simulink model "ABS_Simulink_Model"  (R2023b)
settings: Solver=VariableStepAuto  StartTime=0.0  StopTime=20  RelTol=1e-3
undefined symbols (not defined in the file): A, B, Brake_factor, C, Ch, D, g, I, mv, Rh, Rw, v0
libraries: slpidlib x1
settings Model: Creator=C837312043  LastModifiedBy=C837312043

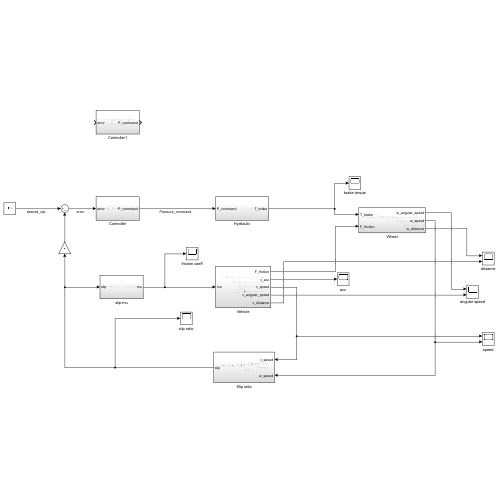
[thumbnail: Simulink's stored preview of the top-level diagram]
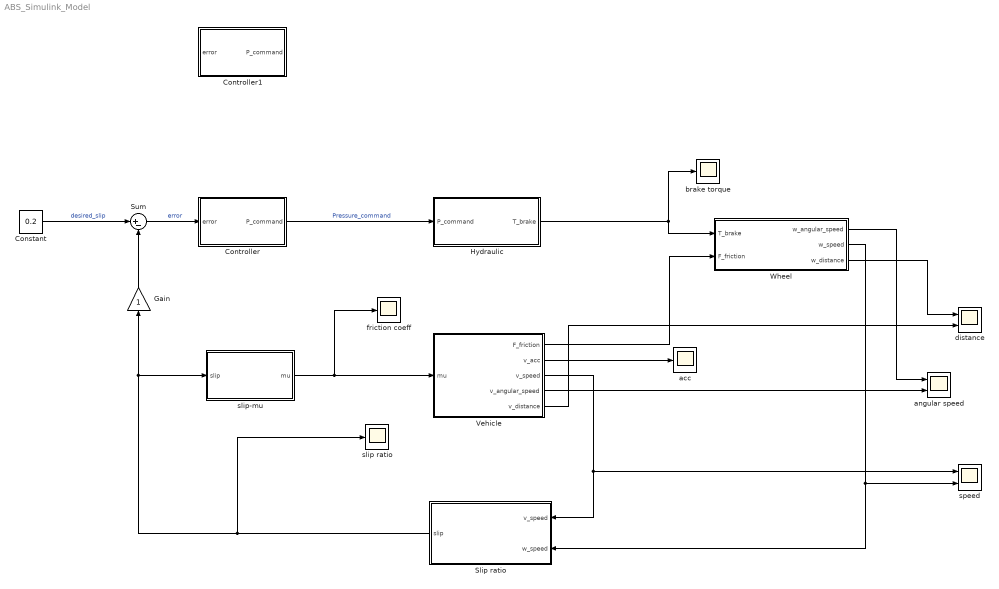
== system ABS_Simulink_Model ==
  Constant : Constant  Value=0.2
  Controller : Subsystem
  Controller1 : Subsystem
  Gain : Gain
  Hydraulic : Subsystem
  Slip ratio : Subsystem
  Sum : Sum  Inputs=|+-
  Vehicle : Subsystem
  Wheel : Subsystem
  acc : Scope
  angular speed : Scope  NumInputPorts=2
  brake torque : Scope
  distance : Scope  NumInputPorts=2
  friction coeff : Scope
  slip ratio : Scope
  slip-mu : Subsystem
  speed : Scope  NumInputPorts=2
  wires:
  Vehicle/1(F_friction) -> Wheel/2(F_friction)
  Wheel/2(w_speed) -> Slip ratio/2(w_speed), speed/2
  Vehicle/3(v_speed) -> speed/1, Slip ratio/1(v_speed)
  Slip ratio/1(slip) -> slip ratio/1, slip-mu/1(slip), Gain/1
  Constant/1 -> Sum/1  "desired_slip"
  Sum/1 -> Controller/1(error)  "error"
  Controller/1(P_command) -> Hydraulic/1(P_command)  "Pressure_command"
  slip-mu/1(mu) -> friction coeff/1, Vehicle/1(mu)
  Hydraulic/1(T_brake) -> brake torque/1, Wheel/1(T_brake)
  Gain/1 -> Sum/2
  Vehicle/2(v_acc) -> acc/1
  Vehicle/4(v_angular_speed) -> angular speed/2
  Wheel/1(w_angular_speed) -> angular speed/1
  Wheel/3(w_distance) -> distance/1
  Vehicle/5(v_distance) -> distance/2

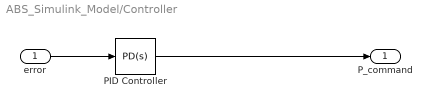
== system ABS_Simulink_Model/Controller ==
  error : Inport
  PID Controller : slpidlib/PID Controller  Controller=PD  Form=Parallel  TimeDomain=Continuous-time  UseExternalTs=off  SampleTime=-1  IntegratorMethod=Forward Euler  FilterMethod=Forward Euler  ControllerParametersSource=internal  P=100  I=50  UseKiTs=off  D=0  N=100  UseFilter=on  TunerSelectOption=Transfer Function Based (PID Tuner App)  InitialConditionSource=internal  InitialConditionForIntegrator=0  InitialConditionForFilter=0  DifferentiatorICPrevScaledInput=0  ExternalReset=none  TrackingMode=off  Kt=1  LimitOutput=off  SatLimitsSource=internal  UpperSaturationLimit=inf  LowerSaturationLimit=-inf  LinearizeAsGain=on  AntiWindupMode=none  Kb=1  LimitIntegrator=off  UpperIntegratorSaturationLimit=inf  LowerIntegratorSaturationLimit=-inf  POutMin=[]  POutMax=[]  IOutMin=[]  IOutMax=[]  DOutMin=[]  DOutMax=[]  NOutMin=[]  NOutMax=[]  SumOutMin=[]  SumOutMax=[]  SaturationOutMin=[]  SaturationOutMax=[]  PParamMin=[]  PParamMax=[]  IParamMin=[]  IParamMax=[]  DParamMin=[]  DParamMax=[]  NParamMin=[]  NParamMax=[]  KbParamMin=[]  KbParamMax=[]  KtParamMin=[]  KtParamMax=[]  KbOutMin=[]  KbOutMax=[]  KtOutMin=[]  KtOutMax=[]  IntegratorOutMin=[]  IntegratorOutMax=[]  FilterOutMin=[]  FilterOutMax=[]  SumI1OutMin=[]  SumI1OutMax=[]  SumI2OutMin=[]  SumI2OutMax=[]  SumI3OutMin=[]  SumI3OutMax=[]  SumI4OutMin=[]  SumI4OutMax=[]  SumDOutMin=[]  SumDOutMax=[]  DifferentiatorOutMin=[]  DifferentiatorOutMax=[]  FilterDiffOutCoefMin=[]  FilterDiffOutCoefMax=[]  ReciprocalOutMin=[]  ReciprocalOutMax=[]  SumDenOutMin=[]  SumDenOutMax=[]  SumNumOutMin=[]  SumNumOutMax=[]  DivideOutMin=[]  DivideOutMax=[]  UdiffTsProdOutMin=[]  UdiffTsProdOutMax=[]  NTsProdOutMin=[]  NTsProdOutMax=[]  UintegralTsProdOutMin=[]  UintegralTsProdOutMax=[]  UngainTsProdOutMin=[]  UngainTsProdOutMax=[]  ClampingZeroOutDataTypeStr=Inherit: Inherit via back propagation  ClampingZeroOutMin=[]  ClampingZeroOutMax=[]  FilterDenConstantOutDataTypeStr=Inherit: Inherit via back propagation  FilterDenConstantOutMin=[]  FilterDenConstantOutMax=[]  PCopyOutDataTypeStr=Inherit: Inherit via back propagation  PCopyOutMin=[]  PCopyOutMax=[]  NCopyOutDataTypeStr=Inherit: Inherit via back propagation  NCopyOutMin=[]  NCopyOutMax=[]  IntegratorContinuousStateAttributes=''  IntegratorStateMustResolveToSignalObject=off  IntegratorRTWStateStorageClass=Auto  FilterContinuousStateAttributes=''  FilterStateMustResolveToSignalObject=off  FilterRTWStateStorageClass=Auto  ParallelPVariant=InternalParameters  IdealPVariant=Disabled  IVariant=Disabled  DVariant=InternalParameters  IntegratorVariant=Disabled  SatVariant=Disabled  AWVariant=Disabled  PCopyVariant=Disabled  TRVariant=Disabled  FdbkBlocksVariant=Forward  IdealPFdbkVariant=Disabled  SatFdbkVariant=Disabled  DerivativeFilterVariant=ContFilter  NVariant=InternalParameters  NCopyVariant=Disabled  FilterICVariant=InternalICsFilter  IntegratorICVariant=Disabled  ExternalResetVariant=Disabled  TRSumVariant=Passthrough  SumFdbkVariant=Disabled  SumVariant=Sum_PD  TsampFilterVariant=InternalTs  TsampNgainVariant=Passthrough  TsampIntegralVariant=Disabled_SignalSpec  ExternalSaturationOutDataTypeStr=Inherit: Same as second input
  P_command : Outport
  wires:
  PID Controller/1 -> P_command/1
  error/1 -> PID Controller/1

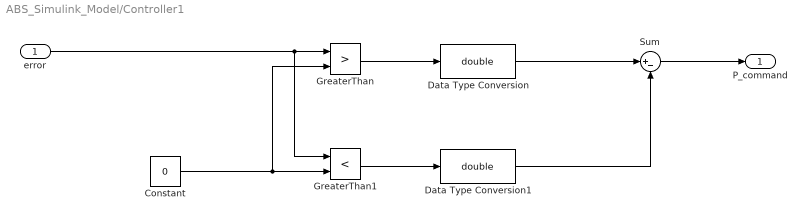
== system ABS_Simulink_Model/Controller1 ==
  error : Inport
  Constant : Constant  Value=0
  Data Type Conversion : DataTypeConversion  OutDataTypeStr=double  SaturateOnIntegerOverflow=off
  Data Type Conversion1 : DataTypeConversion  OutDataTypeStr=double  SaturateOnIntegerOverflow=off
  GreaterThan : RelationalOperator  Operator=>  OutDataTypeStr=boolean  RndMeth=Simplest  InputSameDT=off
  GreaterThan1 : RelationalOperator  Operator=<  OutDataTypeStr=boolean  RndMeth=Simplest  InputSameDT=off
  Sum : Sum  Inputs=|+-
  P_command : Outport
  wires:
  Data Type Conversion1/1 -> Sum/2
  Sum/1 -> P_command/1
  Data Type Conversion/1 -> Sum/1
  GreaterThan1/1 -> Data Type Conversion1/1
  GreaterThan/1 -> Data Type Conversion/1
  Constant/1 -> GreaterThan/2, GreaterThan1/2
  error/1 -> GreaterThan1/1, GreaterThan/1

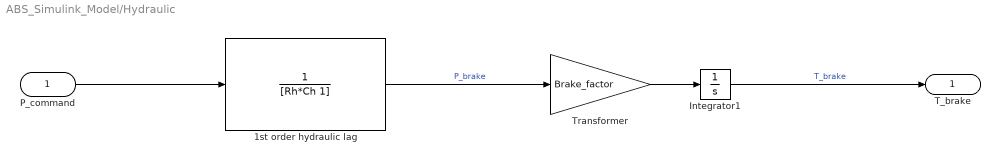
== system ABS_Simulink_Model/Hydraulic ==
  P_command : Inport
  1st order hydraulic lag : TransferFcn  Denominator=[Rh*Ch 1]
  Integrator1 : Integrator  LimitOutput=on  UpperSaturationLimit=2000  LowerSaturationLimit=0
  Transformer : Gain  Gain=Brake_factor
  T_brake : Outport
  wires:
  P_command/1 -> 1st order hydraulic lag/1
  1st order hydraulic lag/1 -> Transformer/1  "P_brake"
  Transformer/1 -> Integrator1/1
  Integrator1/1 -> T_brake/1  "T_brake"

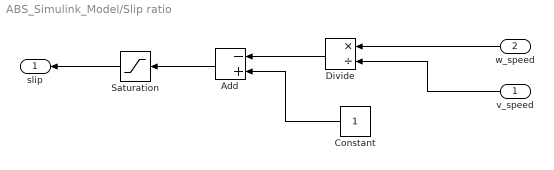
== system ABS_Simulink_Model/Slip ratio ==
  v_speed : Inport
  w_speed : Inport  Port=2
  Add : Sum  Inputs=-+
  Constant : Constant
  Divide : Product  Inputs=*/
  Saturation : Saturate  UpperLimit=1  LowerLimit=0
  slip : Outport
  wires:
  Divide/1 -> Add/1
  w_speed/1 -> Divide/1
  Constant/1 -> Add/2
  Add/1 -> Saturation/1
  Saturation/1 -> slip/1
  v_speed/1 -> Divide/2

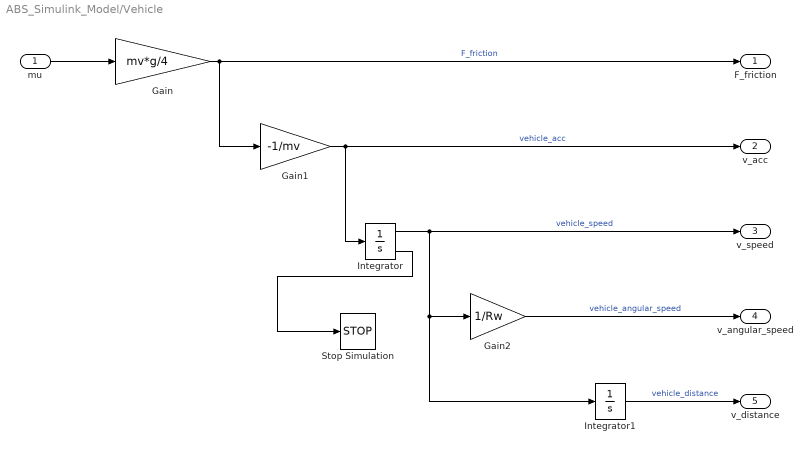
== system ABS_Simulink_Model/Vehicle ==
  mu : Inport
  Gain : Gain  Gain=mv*g/4
  Gain1 : Gain  Gain=-1/mv
  Gain2 : Gain  Gain=1/Rw
  Integrator : Integrator  InitialCondition=v0  LimitOutput=on  UpperSaturationLimit=1000  LowerSaturationLimit=0  ShowSaturationPort=on
  Integrator1 : Integrator
  Stop Simulation : Stop
  F_friction : Outport
  v_acc : Outport  Port=2
  v_speed : Outport  Port=3
  v_angular_speed : Outport  Port=4
  v_distance : Outport  Port=5
  wires:
  mu/1 -> Gain/1
  Integrator1/1 -> v_distance/1  "vehicle_distance"
  Gain1/1 -> v_acc/1, Integrator/1  "vehicle_acc"
  Gain2/1 -> v_angular_speed/1  "vehicle_angular_speed"
  Integrator/1 -> v_speed/1, Gain2/1, Integrator1/1  "vehicle_speed"
  Gain/1 -> F_friction/1, Gain1/1  "F_friction"
  Integrator/2 -> Stop Simulation/1

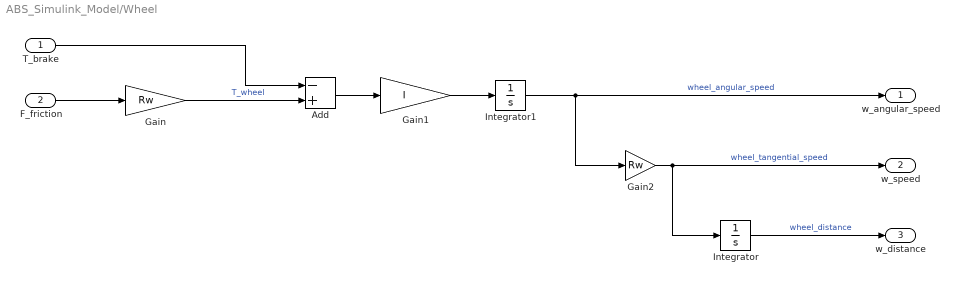
== system ABS_Simulink_Model/Wheel ==
  T_brake : Inport
  F_friction : Inport  Port=2
  Add : Sum  Inputs=-+
  Gain : Gain  Gain=Rw
  Gain1 : Gain  Gain=I
  Gain2 : Gain  Gain=Rw
  Integrator : Integrator
  Integrator1 : Integrator  InitialCondition=v0/Rw  LimitOutput=on  UpperSaturationLimit=1000  LowerSaturationLimit=0
  w_angular_speed : Outport
  w_speed : Outport  Port=2
  w_distance : Outport  Port=3
  wires:
  Gain/1 -> Add/2  "T_wheel"
  F_friction/1 -> Gain/1
  Gain1/1 -> Integrator1/1
  T_brake/1 -> Add/1
  Gain2/1 -> w_speed/1, Integrator/1  "wheel_tangential_speed"
  Add/1 -> Gain1/1
  Integrator/1 -> w_distance/1  "wheel_distance"
  Integrator1/1 -> w_angular_speed/1, Gain2/1  "wheel_angular_speed"

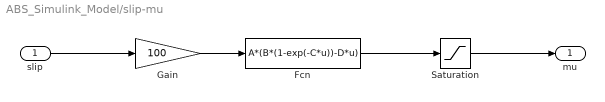
== system ABS_Simulink_Model/slip-mu ==
  slip : Inport
  Fcn : Fcn  Expr=A*(B*(1-exp(-C*u))-D*u)
  Gain : Gain  Gain=100
  Saturation : Saturate  UpperLimit=1  LowerLimit=0
  mu : Outport
  wires:
  slip/1 -> Gain/1
  Fcn/1 -> Saturation/1
  Gain/1 -> Fcn/1
  Saturation/1 -> mu/1
